simulink model "momentumBasedFlight"  (R2023b)
settings: Solver=VariableStepAuto  StartTime=0.0  StopTime=Config.simulationTime  RelTol=1e-3
InitFcn:
  | cd(fileparts(which(bdroot)));
  | initMomentumBasedFlight;
StopFcn:
  | cd(fileparts(which(bdroot)));
  | stopMomentumBasedFlight;
undefined symbols (not defined in the file or in its folder): aero_config, biasVectorConstraint_feet, Config, confVisualizer, ConstraintMatrix_feet, DiscIntNeverNeededParam, frameNames, Frames, jets_config, robot_config
libraries: WBToolboxLibrary x82, momentum_flight_control_v1 x1, deeplib x1, mwbs_robotDynamicsWithContacts_lib x1
(part 3 of 3)

== system momentumBasedFlight/iRonCub/Forward Dynamics/jetsDyn/Simulink Function2 ==
  simFunc_getWorldTransformJet3Frame : TriggerPort  TriggerType=function-call  IsSimulinkFunction=on  FunctionName=simFunc_getWorldTransformJet3Frame  FunctionVisibility=scoped  VariantControl=(inherit)
  ForwardKinematics : WBToolboxLibrary/Model/Kinematics/ForwardKinematics  frameName=Frames.JET3_FRAME
      settings: SourceProductName=WholeBodyToolbox
  basePose : ArgIn  DisableCoverage=on  PortDimensions=[4,4]  ArgumentName=basePose
  jointPosition : ArgIn  Port=2  PortDimensions=[robot_config.N_DOF,1]  ArgumentName=jointPosition
  w_H_jet3Frame : ArgOut  DisableCoverage=on  PortDimensions=[4,4]  ArgumentName=w_H_jet3Frame
  wires:
  ForwardKinematics/1 -> w_H_jet3Frame/1
  jointPosition/1 -> ForwardKinematics/2
  basePose/1 -> ForwardKinematics/1

== system momentumBasedFlight/iRonCub/Forward Dynamics/jetsDyn/Simulink Function3 ==
  simFunc_getWorldTransformJet4Frame : TriggerPort  TriggerType=function-call  IsSimulinkFunction=on  FunctionName=simFunc_getWorldTransformJet4Frame  FunctionVisibility=scoped  VariantControl=(inherit)
  ForwardKinematics : WBToolboxLibrary/Model/Kinematics/ForwardKinematics  frameName=Frames.JET4_FRAME
      settings: SourceProductName=WholeBodyToolbox
  basePose : ArgIn  DisableCoverage=on  PortDimensions=[4,4]  ArgumentName=basePose
  jointPosition : ArgIn  Port=2  PortDimensions=[robot_config.N_DOF,1]  ArgumentName=jointPosition
  w_H_jet4Frame : ArgOut  DisableCoverage=on  PortDimensions=[4,4]  ArgumentName=w_H_jet4Frame
  wires:
  basePose/1 -> ForwardKinematics/1
  jointPosition/1 -> ForwardKinematics/2
  ForwardKinematics/1 -> w_H_jet4Frame/1

== system momentumBasedFlight/iRonCub/Forward Dynamics/jetsDyn/Simulink Function4 ==
  simFunc_getFrameFreeFloatingJacobianJet2Frame : TriggerPort  TriggerType=function-call  IsSimulinkFunction=on  FunctionName=simFunc_getFrameFreeFloatingJacobianJet2Frame  FunctionVisibility=scoped  VariantControl=(inherit)
  Jacobian Left Foot : WBToolboxLibrary/Model/Jacobians/Jacobian  frameName=Frames.JET2_FRAME
      settings: SourceProductName=WholeBodyToolbox
  basePose : ArgIn  DisableCoverage=on  PortDimensions=[4,4]  ArgumentName=basePose
  jointPosition : ArgIn  Port=2  PortDimensions=[robot_config.N_DOF,1]  ArgumentName=jointPosition
  jacobian : ArgOut  DisableCoverage=on  PortDimensions=[6,6+robot_config.N_DOF]  ArgumentName=jacobian
  wires:
  Jacobian Left Foot/1 -> jacobian/1
  jointPosition/1 -> Jacobian Left Foot/2
  basePose/1 -> Jacobian Left Foot/1

== system momentumBasedFlight/iRonCub/Forward Dynamics/jetsDyn/Simulink Function5 ==
  simFunc_getFrameFreeFloatingJacobianJet3Frame : TriggerPort  TriggerType=function-call  IsSimulinkFunction=on  FunctionName=simFunc_getFrameFreeFloatingJacobianJet3Frame  FunctionVisibility=scoped  VariantControl=(inherit)
  Jacobian Left Foot : WBToolboxLibrary/Model/Jacobians/Jacobian  frameName=Frames.JET3_FRAME
      settings: SourceProductName=WholeBodyToolbox
  basePose : ArgIn  DisableCoverage=on  PortDimensions=[4,4]  ArgumentName=basePose
  jointPosition : ArgIn  Port=2  PortDimensions=[robot_config.N_DOF,1]  ArgumentName=jointPosition
  jacobian : ArgOut  DisableCoverage=on  PortDimensions=[6,6+robot_config.N_DOF]  ArgumentName=jacobian
  wires:
  Jacobian Left Foot/1 -> jacobian/1
  jointPosition/1 -> Jacobian Left Foot/2
  basePose/1 -> Jacobian Left Foot/1

== system momentumBasedFlight/iRonCub/Forward Dynamics/jetsDyn/Simulink Function6 ==
  simFunc_getFrameFreeFloatingJacobianJet4Frame : TriggerPort  TriggerType=function-call  IsSimulinkFunction=on  FunctionName=simFunc_getFrameFreeFloatingJacobianJet4Frame  FunctionVisibility=scoped  VariantControl=(inherit)
  Jacobian Left Foot : WBToolboxLibrary/Model/Jacobians/Jacobian  frameName=Frames.JET4_FRAME
      settings: SourceProductName=WholeBodyToolbox
  basePose : ArgIn  DisableCoverage=on  PortDimensions=[4,4]  ArgumentName=basePose
  jointPosition : ArgIn  Port=2  PortDimensions=[robot_config.N_DOF,1]  ArgumentName=jointPosition
  jacobian : ArgOut  DisableCoverage=on  PortDimensions=[6,6+robot_config.N_DOF]  ArgumentName=jacobian
  wires:
  Jacobian Left Foot/1 -> jacobian/1
  jointPosition/1 -> Jacobian Left Foot/2
  basePose/1 -> Jacobian Left Foot/1

== system momentumBasedFlight/iRonCub/Forward Dynamics/jetsDyn/Simulink Function7 ==
  simFunc_getWorldTransformJet1Frame : TriggerPort  TriggerType=function-call  IsSimulinkFunction=on  FunctionName=simFunc_getWorldTransformJet1Frame  FunctionVisibility=scoped  VariantControl=(inherit)
  ForwardKinematics : WBToolboxLibrary/Model/Kinematics/ForwardKinematics  frameName=Frames.JET1_FRAME
      settings: SourceProductName=WholeBodyToolbox
  basePose : ArgIn  DisableCoverage=on  PortDimensions=[4,4]  ArgumentName=basePose
  jointPosition : ArgIn  Port=2  PortDimensions=[robot_config.N_DOF,1]  ArgumentName=jointPosition
  w_H_jet1Frame : ArgOut  DisableCoverage=on  PortDimensions=[4,4]  ArgumentName=w_H_jet1Frame
  wires:
  basePose/1 -> ForwardKinematics/1
  jointPosition/1 -> ForwardKinematics/2
  ForwardKinematics/1 -> w_H_jet1Frame/1

== system momentumBasedFlight/FLIGHT CONTROLLER (CORE) V3.0/Flight Controller RAL-HUMANOIDS V3.0/Joint Torque Control for Flying/QP torqueControl/QP torqueControl - balancing ==
  H : Inport
  g : Inport  Port=2
  ub : Inport  Port=3
  lb : Inport  Port=4
  AEq : Inport  Port=5
  lbEq : Inport  Port=6
  ubEq : Inport  Port=7
  Enable : EnablePort
  Combine Bounds and Inequalities : MATLAB Function  TreatAsAtomicUnit=on
  MatchSignalSizes : WBToolboxLibrary/Utilities/MatchSignalSizes
      settings: SourceProductName=WholeBodyToolbox
  QP balancing-torqueControl : WBToolboxLibrary/Utilities/QP  lbA=on  ubA=on  lb=off  ub=off  computeObjVal=off  stopIfFails=off
      settings: SourceProductName=WholeBodyToolbox
  QPStatus_balancing : Outport  VectorParamsAs1DForOutWhenUnconnected=off
  QPOutput_balancing : Outport  Port=2  VectorParamsAs1DForOutWhenUnconnected=off
  wires:
  Combine Bounds and Inequalities/3(ubEq_combined) -> QP balancing-torqueControl/5
  Combine Bounds and Inequalities/2(lbEq_combined) -> QP balancing-torqueControl/4
  Combine Bounds and Inequalities/1(AEq_combined) -> QP balancing-torqueControl/3
  ub/1 -> Combine Bounds and Inequalities/5(ub)
  lb/1 -> Combine Bounds and Inequalities/4(lb)
  ubEq/1 -> Combine Bounds and Inequalities/3(ubEq)
  lbEq/1 -> Combine Bounds and Inequalities/2(lbEq)
  AEq/1 -> Combine Bounds and Inequalities/1(AEq)
  g/1 -> QP balancing-torqueControl/2, MatchSignalSizes/1
  H/1 -> QP balancing-torqueControl/1
  QP balancing-torqueControl/1 -> MatchSignalSizes/2
  MatchSignalSizes/1 -> QPOutput_balancing/1
  QP balancing-torqueControl/2 -> QPStatus_balancing/1

== system momentumBasedFlight/FLIGHT CONTROLLER (CORE) V3.0/Flight Controller RAL-HUMANOIDS V3.0/Joint Torque Control for Flying/QP torqueControl/QP torqueControl - flight ==
  H : Inport
  g : Inport  Port=2
  ub : Inport  Port=3
  lb : Inport  Port=4
  Enable : EnablePort
  Constant : Constant  Value=eye(Config.N_DOF)
  MatchSignalSizes : WBToolboxLibrary/Utilities/MatchSignalSizes
      settings: SourceProductName=WholeBodyToolbox
  QP flight-torqueControl : WBToolboxLibrary/Utilities/QP  lbA=on  ubA=on  lb=off  ub=off  computeObjVal=off  stopIfFails=off
      settings: SourceProductName=WholeBodyToolbox
  QPStatus_flight : Outport  VectorParamsAs1DForOutWhenUnconnected=off
  QPOutput_flight : Outport  Port=2  VectorParamsAs1DForOutWhenUnconnected=off
  wires:
  ub/1 -> QP flight-torqueControl/5
  g/1 -> MatchSignalSizes/1, QP flight-torqueControl/2
  H/1 -> QP flight-torqueControl/1
  QP flight-torqueControl/1 -> MatchSignalSizes/2
  MatchSignalSizes/1 -> QPOutput_flight/1
  lb/1 -> QP flight-torqueControl/4
  QP flight-torqueControl/2 -> QPStatus_flight/1
  Constant/1 -> QP flight-torqueControl/3

== system momentumBasedFlight/FLIGHT CONTROLLER (CORE) V3.0/Flight Controller RAL-HUMANOIDS V3.0/Joint Torque Control for Flying/QP torqueControl/Select QP torqueControl Output ==
  QPStatus_balancing : Inport
  QPOutput_balancing : Inport  Port=2
  feetContactIsActive : Inport  Port=3
  QPStatus_flight : Inport  Port=4
  QPOutput_flight : Inport  Port=5
  Demux : Demux  Outputs=[12;Config.N_DOF]
  Switch : Switch  Criteria=u2 > Threshold  SaturateOnIntegerOverflow=off  InputSameDT=off
  Switch1 : Switch  Criteria=u2 > Threshold  SaturateOnIntegerOverflow=off  InputSameDT=off
  contactForces_QP : Terminator
  jointTorques_star : Outport  VectorParamsAs1DForOutWhenUnconnected=off
  exitFlagQP_torqueControl : Outport  Port=2  VectorParamsAs1DForOutWhenUnconnected=off
  wires:
  Demux/2 -> Switch1/1
  Demux/1 -> contactForces_QP/1
  QPOutput_flight/1 -> Switch1/3
  QPOutput_balancing/1 -> Demux/1
  Switch/1 -> exitFlagQP_torqueControl/1
  QPStatus_flight/1 -> Switch/3
  QPStatus_balancing/1 -> Switch/1
  feetContactIsActive/1 -> Switch/2, Switch1/2
  Switch1/1 -> jointTorques_star/1

== system momentumBasedFlight/FLIGHT CONTROLLER (CORE) V3.0/Flight Controller RAL-HUMANOIDS V3.0/Momentum Control for Flying/QP Solver and Integrate Contact Forces Derivative/Integrate the Contact Forces Derivative ==
  contactForcesDot_star : Inport
  contactForces : Inport  Port=2
  feetContactIsActive : Inport  Port=3
  Discrete-Time Integrator1 : DiscreteIntegrator  ExternalReset=either  InitialConditionSource=external  InitialCondition=zeros(6,1)  SampleTime=Config.tStep  ICPrevOutput=DiscIntNeverNeededParam  ICPrevScaledInput=DiscIntNeverNeededParam
  Select Integrator Initial Condition : MATLAB Function  TreatAsAtomicUnit=on
  deadZone : Subsystem
  contactForces_star : Outport  VectorParamsAs1DForOutWhenUnconnected=off
  tag scope: contactForcesDot_star=global
  wires:
  Select Integrator Initial Condition/1(contactForces_0) -> Discrete-Time Integrator1/3
  feetContactIsActive/1 -> Discrete-Time Integrator1/2, Select Integrator Initial Condition/1(feetContactIsActive)
  contactForces/1 -> Select Integrator Initial Condition/2(contactForces)
  deadZone/1(u_cut) -> Discrete-Time Integrator1/1
  contactForcesDot_star/1 -> [contactForcesDot_star], deadZone/1(u)
  Discrete-Time Integrator1/1 -> contactForces_star/1

== system momentumBasedFlight/FLIGHT CONTROLLER (CORE) V3.0/Flight Controller RAL-HUMANOIDS V3.0/Momentum Control for Flying/QP Solver and Integrate Contact Forces Derivative/QP momentumControl ==
  HessianMatrixQP : Inport
  gVectorQP : Inport  Port=2
  lowerBoundQP : Inport  Port=3
  upperBoundQP : Inport  Port=4
  feetContactIsActive : Inport  Port=5
  NOT : Logic  Operator=NOT  IconShape=distinctive  AllPortsSameDT=off  OutDataTypeStr=boolean
  Process QP Inputs Momentum Control : MATLAB Function  TreatAsAtomicUnit=on
  QP momentumControl - balancing : Subsystem  TreatAsAtomicUnit=on
  QP momentumControl - flight : Subsystem  TreatAsAtomicUnit=on
  Select QP momentumControl Output : Subsystem
  jetsIntensitiesDot_star : Outport  VectorParamsAs1DForOutWhenUnconnected=off
  contactForcesDot_star : Outport  Port=2  VectorParamsAs1DForOutWhenUnconnected=off
  jointVel_star : Outport  Port=3  VectorParamsAs1DForOutWhenUnconnected=off
  exitFlagQP_momentumControl : Outport  Port=4  VectorParamsAs1DForOutWhenUnconnected=off
  wires:
  QP momentumControl - flight/2(QPOutput_flight) -> Select QP momentumControl Output/5(QPOutput_flight)
  QP momentumControl - flight/1(QPStatus_flight) -> Select QP momentumControl Output/4(QPStatus_flight)
  QP momentumControl - balancing/2(QPOutput_balancing) -> Select QP momentumControl Output/2(QPOutput_balancing)
  QP momentumControl - balancing/1(QPStatus_balancing) -> Select QP momentumControl Output/1(QPStatus_balancing)
  Select QP momentumControl Output/4(exitFlagQP_momentumControl) -> exitFlagQP_momentumControl/1
  NOT/1 -> QP momentumControl - flight/Enable
  Process QP Inputs Momentum Control/8(lb_flight) -> QP momentumControl - flight/4(lb)
  Process QP Inputs Momentum Control/7(ub_flight) -> QP momentumControl - flight/3(ub)
  Process QP Inputs Momentum Control/4(lb_balancing) -> QP momentumControl - balancing/4(lb)
  Process QP Inputs Momentum Control/3(ub_balancing) -> QP momentumControl - balancing/3(ub)
  Process QP Inputs Momentum Control/6(g_flight) -> QP momentumControl - flight/2(g)
  Process QP Inputs Momentum Control/5(H_flight) -> QP momentumControl - flight/1(H)
  Process QP Inputs Momentum Control/2(g_balancing) -> QP momentumControl - balancing/2(g)
  Process QP Inputs Momentum Control/1(H_balancing) -> QP momentumControl - balancing/1(H)
  Select QP momentumControl Output/2(contactForcesDot_star) -> contactForcesDot_star/1
  Select QP momentumControl Output/3(jointVel_star) -> jointVel_star/1
  Select QP momentumControl Output/1(jetsIntensitiesDot_star) -> jetsIntensitiesDot_star/1
  HessianMatrixQP/1 -> Process QP Inputs Momentum Control/1(HessianMatrixQP)
  upperBoundQP/1 -> Process QP Inputs Momentum Control/4(upperBoundQP)
  feetContactIsActive/1 -> QP momentumControl - balancing/Enable, NOT/1, Select QP momentumControl Output/3(feetContactIsActive)
  lowerBoundQP/1 -> Process QP Inputs Momentum Control/3(lowerBoundQP)
  gVectorQP/1 -> Process QP Inputs Momentum Control/2(gVectorQP)

== system momentumBasedFlight/FLIGHT CONTROLLER (CORE) V3.0/Flight Controller RAL-HUMANOIDS V3.0/Momentum Control for Flying/QP Solver and Integrate Contact Forces Derivative/Integrate the Contact Forces Derivative/deadZone ==
  u : Inport
  Constant : Constant  Value=Config.sat.deadZoneThreshold
  Deadzone Function : MATLAB Function  TreatAsAtomicUnit=on
  u_cut : Outport  VectorParamsAs1DForOutWhenUnconnected=off
  wires:
  Constant/1 -> Deadzone Function/2(thr)
  u/1 -> Deadzone Function/1(u)
  Deadzone Function/1(y) -> u_cut/1

== system momentumBasedFlight/FLIGHT CONTROLLER (CORE) V3.0/Flight Controller RAL-HUMANOIDS V3.0/Momentum Control for Flying/QP Solver and Integrate Contact Forces Derivative/QP momentumControl/QP momentumControl - balancing ==
  H : Inport
  g : Inport  Port=2
  ub : Inport  Port=3
  lb : Inport  Port=4
  Enable : EnablePort
  Constant : Constant  Value=eye(Config.N_DOF + 12 + 4)
  MatchSignalSizes : WBToolboxLibrary/Utilities/MatchSignalSizes
      settings: SourceProductName=WholeBodyToolbox
  QP : WBToolboxLibrary/Utilities/QP  lbA=on  ubA=on  lb=off  ub=off  computeObjVal=off  stopIfFails=off
      settings: SourceProductName=WholeBodyToolbox
  QPStatus_balancing : Outport  VectorParamsAs1DForOutWhenUnconnected=off
  QPOutput_balancing : Outport  Port=2  VectorParamsAs1DForOutWhenUnconnected=off
  wires:
  ub/1 -> QP/5
  QP/1 -> MatchSignalSizes/2
  MatchSignalSizes/1 -> QPOutput_balancing/1
  QP/2 -> QPStatus_balancing/1
  H/1 -> QP/1
  g/1 -> MatchSignalSizes/1, QP/2
  lb/1 -> QP/4
  Constant/1 -> QP/3

== system momentumBasedFlight/FLIGHT CONTROLLER (CORE) V3.0/Flight Controller RAL-HUMANOIDS V3.0/Momentum Control for Flying/QP Solver and Integrate Contact Forces Derivative/QP momentumControl/QP momentumControl - flight ==
  H : Inport
  g : Inport  Port=2
  ub : Inport  Port=3
  lb : Inport  Port=4
  Enable : EnablePort
  Constant : Constant  Value=eye(Config.N_DOF + 4)
  MatchSignalSizes : WBToolboxLibrary/Utilities/MatchSignalSizes
      settings: SourceProductName=WholeBodyToolbox
  QP flight-momentumControl : WBToolboxLibrary/Utilities/QP  lbA=on  ubA=on  lb=off  ub=off  computeObjVal=off  stopIfFails=off
      settings: SourceProductName=WholeBodyToolbox
  QPStatus_flight : Outport  VectorParamsAs1DForOutWhenUnconnected=off
  QPOutput_flight : Outport  Port=2  VectorParamsAs1DForOutWhenUnconnected=off
  wires:
  ub/1 -> QP flight-momentumControl/5
  g/1 -> MatchSignalSizes/1, QP flight-momentumControl/2
  H/1 -> QP flight-momentumControl/1
  QP flight-momentumControl/1 -> MatchSignalSizes/2
  MatchSignalSizes/1 -> QPOutput_flight/1
  lb/1 -> QP flight-momentumControl/4
  QP flight-momentumControl/2 -> QPStatus_flight/1
  Constant/1 -> QP flight-momentumControl/3

== system momentumBasedFlight/FLIGHT CONTROLLER (CORE) V3.0/Flight Controller RAL-HUMANOIDS V3.0/Momentum Control for Flying/QP Solver and Integrate Contact Forces Derivative/QP momentumControl/Select QP momentumControl Output ==
  QPStatus_balancing : Inport
  QPOutput_balancing : Inport  Port=2
  feetContactIsActive : Inport  Port=3
  QPStatus_flight : Inport  Port=4
  QPOutput_flight : Inport  Port=5
  Constant : Constant  Value=zeros(12,1)
  Demux : Demux  Outputs=[4;12;Config.N_DOF]
  Demux1 : Demux  Outputs=[4;Config.N_DOF]
  Switch{,1..3} (4 alike) : Switch  Criteria=u2 > Threshold  SaturateOnIntegerOverflow=off  InputSameDT=off
  jetsIntensitiesDot_star : Outport  VectorParamsAs1DForOutWhenUnconnected=off
  contactForcesDot_star : Outport  Port=2  VectorParamsAs1DForOutWhenUnconnected=off
  jointVel_star : Outport  Port=3  VectorParamsAs1DForOutWhenUnconnected=off
  exitFlagQP_momentumControl : Outport  Port=4  VectorParamsAs1DForOutWhenUnconnected=off
  wires:
  Demux1/2 -> Switch3/3
  Demux/3 -> Switch3/1
  Constant/1 -> Switch2/3
  Demux/2 -> Switch2/1
  Demux1/1 -> Switch1/3
  Demux/1 -> Switch1/1
  QPOutput_flight/1 -> Demux1/1
  QPOutput_balancing/1 -> Demux/1
  Switch/1 -> exitFlagQP_momentumControl/1
  QPStatus_flight/1 -> Switch/3
  QPStatus_balancing/1 -> Switch/1
  feetContactIsActive/1 -> Switch/2, Switch1/2, Switch2/2, Switch3/2
  Switch3/1 -> jointVel_star/1
  Switch1/1 -> jetsIntensitiesDot_star/1
  Switch2/1 -> contactForcesDot_star/1

== matlab function momentumBasedFlight/FLIGHT CONTROLLER (CORE) V3.0/Jets Control/Feedback linearization/MATLAB Function ==
  data: jets input; jets_dot input; jets_dot_des input; throttle output size=[4,1]; Config parameter; error output; integral_err input
function [throttle, error]  = fl_jet_control(jets, jets_dot, jets_dot_des, Config, integral_err)

[throttle, error]  = fl_jet_control(jets, jets_dot, jets_dot_des, Config, integral_err);
end

== matlab function momentumBasedFlight/FLIGHT CONTROLLER (CORE) V3.0/Flight Controller RAL-HUMANOIDS V3.0/Joint Torque Control for Flying/QP torqueControl/Process QP Inputs Torque Control ==
  data: HessianMatrixQP input; H_balancing output; gVectorQP input; InequalityConstrMatrix input; biasVectorInequalityConstr input; g_balancing output; ub_balancing output; lb_balancing output; Aeq_balancing output; lbEq_balancing output; ubEq_balancing output; H_flight output; g_flight output; ub_flight output; lb_flight output; jointTorquesSaturation input; Config parameter
function [H_balancing,g_balancing,ub_balancing,lb_balancing,Aeq_balancing,lbEq_balancing,ubEq_balancing, ...
          H_flight,g_flight,ub_flight,lb_flight] = processQPinputTorqueControlFCN ...
                                                       (HessianMatrixQP,gVectorQP,InequalityConstrMatrix, ...
                                                        biasVectorInequalityConstr,jointTorquesSaturation,Config)   
   
[H_balancing,g_balancing,ub_balancing,lb_balancing,Aeq_balancing,lbEq_balancing,ubEq_balancing, ...
          H_flight,g_flight,ub_flight,lb_flight] = iRonCubLib_v1.processQPinputTorqueControl ...
                                                       (HessianMatrixQP,gVectorQP,InequalityConstrMatrix, ...
                                                        biasVectorInequalityConstr,jointTorquesSaturation,Config);     
end

== matlab function momentumBasedFlight/FLIGHT CONTROLLER (CORE) V3.0/Flight Controller RAL-HUMANOIDS V3.0/Joint Torque Control for Flying/QP torqueControl/QP torqueControl - balancing/Combine Bounds and Inequalities ==
  data: AEq input; AEq_combined output; lbEq input; ubEq input; lb input; ub input; lbEq_combined output; ubEq_combined output
function [AEq_combined,lbEq_combined,ubEq_combined] = combineInputBoundsAndInequalitiesQPFCN(AEq,lbEq,ubEq,lb,ub)

   [AEq_combined,lbEq_combined,ubEq_combined] = iRonCubLib_v1.combineInputBoundsAndInequalitiesQP(AEq,lbEq,ubEq,lb,ub);
end

== matlab function momentumBasedFlight/FLIGHT CONTROLLER (CORE) V3.0/Jets Control/extendedKalmanFilter4jets/EKF_jet1/EKF  ==
  data: x input; input input; measurement input; xDot output; P input; Config parameter; Pdot output
function [xDot, Pdot] = extendedKalmanFilterFNC(x, input, measurement, P, Config)

[xDot, Pdot] = extKalmanFilter(x, input, Config.jetC_P100, P, measurement, Config);

== matlab function momentumBasedFlight/FLIGHT CONTROLLER (CORE) V3.0/Flight Controller RAL-HUMANOIDS V3.0/Joint Torque Control for Flying/torqueControlFCN ==
  data: M input; h input; J_jets input; J_LFoot input; J_RFoot input; JDot_LFoot_nu input; JDot_RFoot_nu input; J_aeroForces input; w_H_LFoot input; w_H_RFoot input; matrixOfJetsAxes input; ConstraintsMatrix_feet input; biasVectorConstraint_feet input; jetsIntensities input; stateVel input; jointVel_star input; contactForces_star input; KI_torqueControl input; KP_torqueControl input; feetContactIsActive input; activateEqConstrTorqueControl input; robotIsLanded input; aerodynamic_forces input; jointPos_err input; Hessian output; Config parameter; gradient output; ConstraintMatrix_inequality output; biasVectorConstraint_inequality output; jointVel_err output; aero_config parameter
function [Hessian, gradient, ConstraintMatrix_inequality, biasVectorConstraint_inequality, jointVel_err] =  ... 
             aeroFlyingTorqueControlFCN(M, h, J_jets, J_LFoot, J_RFoot, JDot_LFoot_nu, JDot_RFoot_nu, J_aeroForces, w_H_LFoot, w_H_RFoot, matrixOfJetsAxes, ...
                                        ConstraintsMatrix_feet, biasVectorConstraint_feet, jetsIntensities, stateVel, jointVel_star, contactForces_star, ...
                                        KI_torqueControl, KP_torqueControl, feetContactIsActive, activateEqConstrTorqueControl, robotIsLanded, aerodynamic_forces, jointPos_err, Config, aero_config)
                                      
    [Hessian, gradient, ConstraintMatrix_inequality, biasVectorConstraint_inequality, jointVel_err] =  ... 
        aeroFlyingTorqueControl(M, h, J_jets, J_LFoot, J_RFoot, JDot_LFoot_nu, JDot_RFoot_nu, J_aeroForces, w_H_LFoot, w_H_RFoot, matrixOfJetsAxes, ...
                                ConstraintsMatrix_feet, biasVectorConstraint_feet, jetsIntensities, stateVel, jointVel_star, contactForces_star, ...
                                KI_torqueControl, KP_torqueControl, feetContactIsActive, activateEqConstrTorqueControl, robotIsLanded, aerodynamic_forces, jointPos_err, aero_config, Config);           
end

== matlab function momentumBasedFlight/FLIGHT CONTROLLER (CORE) V3.0/Flight Controller RAL-HUMANOIDS V3.0/Momentum Control for Flying/Momentum Control/Aerodynamic Flying Controller Momentum FCN  ==
  data: jointPos input; w_baseTwist input; jetsIntensities input; J_jets input; J_CoM input; J_LFoot input; J_RFoot input; posCoM input; w_R_b input; w_H_LFoot input; w_H_RFoot input; matrixOfJetsAxes input; matrixOfJetsArms input; matrixOfAeroArms input; J_aeroForces input; w_I_c input; L input; M input; CMM input; pos_vel_acc_jerk_CoM_des input; rot_vel_acc_jerk_base_des input size=[3,6]; jointPos_des input; KP_momentum input; KD_momentum input; KP_postural input; feetContactIsActive input; decreaseMaxFootVerticalForce input; increaseMinFootVerticalForce input; robotIsLanded input; HessianMatrixQP output; gVectorQP output; lowerBoundQP output; upperBoundQP output; L_des output; LDot_estimated output; verifyAngMomAndInertia output; contactForces_hat input; aerodynamic_forces input; Config parameter; velCoM output; aero_config parameter
function [HessianMatrixQP, gVectorQP, lowerBoundQP, upperBoundQP, L_des, LDot_estimated, verifyAngMomAndInertia, velCoM] = ...
             aeroFlyingMomentumControlFCN(jointPos, w_baseTwist, jetsIntensities, J_jets, J_CoM, J_LFoot, J_RFoot, posCoM, w_R_b, w_H_LFoot, w_H_RFoot, ...
                                          matrixOfJetsAxes, matrixOfJetsArms, matrixOfAeroArms, J_aeroForces, w_I_c, L, M, CMM, pos_vel_acc_jerk_CoM_des, ....
                                          rot_vel_acc_jerk_base_des, jointPos_des, KP_momentum, KD_momentum, KP_postural, feetContactIsActive, ...
                                          decreaseMaxFootVerticalForce, increaseMinFootVerticalForce, robotIsLanded, contactForces_hat, aerodynamic_forces, Config, aero_config)
                               
    [HessianMatrixQP, gVectorQP, lowerBoundQP, upperBoundQP, L_des, LDot_estimated, verifyAngMomAndInertia, velCoM] = ...
        aeroFlyingMomentumControl(jointPos, w_baseTwist, jetsIntensities, J_jets, J_CoM, J_LFoot, J_RFoot, posCoM, w_R_b, w_H_LFoot, w_H_RFoot, ...
                                  matrixOfJetsAxes, matrixOfJetsArms, matrixOfAeroArms, J_aeroForces, w_I_c, L, M, CMM, pos_vel_acc_jerk_CoM_des, ....
                                  rot_vel_acc_jerk_base_des, jointPos_des, KP_momentum, KD_momentum, KP_postural, feetContactIsActive, ...
                                  decreaseMaxFootVerticalForce, increaseMinFootVerticalForce, robotIsLanded, contactForces_hat, aerodynamic_forces, aero_config, Config);
end

== matlab function momentumBasedFlight/FLIGHT CONTROLLER (CORE) V3.0/Jets Control/extendedKalmanFilter4jets/EKF_jet1/splitVector ==
  data: x input; x1 output; x2 output
function [x1, x2] = fcn(x)
x1 = x(1);
x2 = x(2);

== matlab function momentumBasedFlight/Visualizer/Task and Base Frame Kinematics/Get RPY error norm ==
  data: rot_err input; rotErr_norm output
function rotErr_norm = normFCN(rot_err)

rotErr_norm = norm(rot_err);

end

== matlab function momentumBasedFlight/FLIGHT CONTROLLER (CORE) V3.0/Flight Controller RAL-HUMANOIDS V3.0/Momentum Control for Flying/QP Solver and Integrate Contact Forces Derivative/Integrate the Contact Forces Derivative/Select Integrator Initial Condition ==
  data: feetContactIsActive input; contactForces input; contactForces_0 output
function contactForces_0 = selectInitContactForcesFCN(feetContactIsActive, contactForces)

    contactForces_0 = iRonCubLib_v1.selectInitContactForces(feetContactIsActive, contactForces);
end

== matlab function momentumBasedFlight/FLIGHT CONTROLLER (CORE) V3.0/Jets Control/extendedKalmanFilter4jets/EKF_jet2/EKF  ==
  data: x input; input input; measurement input; xDot output; P input; Config parameter; Pdot output
function [xDot, Pdot] = extendedKalmanFilterFNC(x, input, measurement, P, Config)

[xDot, Pdot] = extKalmanFilter(x, input, Config.jetC_P100, P, measurement, Config);

== matlab function momentumBasedFlight/FLIGHT CONTROLLER (CORE) V3.0/Dynamics and Kinematics/Kinematic Quantities/Compute Aerodynamic Forces Homogeneous Transform/Aero Transforms ==
  data: w_H_LinkFrames input; posCoM input; matrixOfLinkCoMTransform output; Config parameter; aero_config parameter
function matrixOfLinkCoMTransform = computeMatrixOfLinkCoMTransformFCN(w_H_LinkFrames, posCoM, Config, aero_config)

    matrixOfLinkCoMTransform = computeMatrixOfLinkCoMTransform(w_H_LinkFrames, posCoM, aero_config, Config);
end

== matlab function momentumBasedFlight/FLIGHT CONTROLLER (CORE) V3.0/Get System State/Change Contact Forces Representation/Change Contact Forces Representation ==
  data: contactForces_WBD input; mixed_f_l_sole output; w_R_l_sole input; w_R_r_sole input; mixed_f_r_sole output
function [mixed_f_l_sole, mixed_f_r_sole] = fromBodyFrameToMixed_contactForcesFCN(contactForces_WBD, w_R_l_sole, w_R_r_sole)

    [mixed_f_l_sole, mixed_f_r_sole] = iRonCubLib_v1.fromBodyFrameToMixed_contactForces(contactForces_WBD, w_R_l_sole, w_R_r_sole);
end

== matlab function momentumBasedFlight/Visualizer/Task and Base Frame Kinematics/Get RPY from rotation matrix ==
  data: w_R_b input; rollPitchYaw output
function rollPitchYaw = rollPitchYawFromRotationFCN(w_R_b)

rollPitchYaw = wbc.rollPitchYawFromRotation(w_R_b);

end

== matlab function momentumBasedFlight/Visualizer/Task and Base Frame Kinematics/Get RPY from rotation matrix  ==
  data: w_R_b input; rollPitchYaw output
function rollPitchYaw = rollPitchYawFromRotationFCN(w_R_b)

rollPitchYaw = wbc.rollPitchYawFromRotation(w_R_b);

end

== matlab function momentumBasedFlight/Visualizer/Task and Base Frame Kinematics/MATLAB Function1 ==
  data: RPY_Corr output; rollPitchYaw input
function RPY_Corr = correctYawAngleFCN(rollPitchYaw)

    RPY_Corr = correctYawAngle(rollPitchYaw);

end

== matlab function momentumBasedFlight/FLIGHT CONTROLLER (CORE) V3.0/Jets Control/extendedKalmanFilter4jets/EKF_jet2/splitVector ==
  data: x input; x1 output; x2 output
function [x1, x2] = fcn(x)
x1 = x(1);
x2 = x(2);

== matlab function momentumBasedFlight/FLIGHT CONTROLLER (CORE) V3.0/Jets Control/extendedKalmanFilter4jets/EKF_jet3/EKF  ==
  data: x input; input input; measurement input; xDot output; P input; Config parameter; Pdot output
function [xDot, Pdot] = extendedKalmanFilterFNC(x, input, measurement, P, Config)

[xDot, Pdot] = extKalmanFilter(x, input, Config.jetC_P220, P, measurement, Config);

== matlab function momentumBasedFlight/Visualizer/Task and Base Frame Kinematics/MATLAB Function2 ==
  data: RPY_Corr output; rollPitchYaw input
function RPY_Corr = correctYawAngleFCN(rollPitchYaw)

    RPY_Corr = correctYawAngle(rollPitchYaw);

end

== matlab function momentumBasedFlight/FLIGHT CONTROLLER (CORE) V3.0/Jets Control/extendedKalmanFilter4jets/EKF_jet3/splitVector ==
  data: x input; x1 output; x2 output
function [x1, x2] = fcn(x)
x1 = x(1);
x2 = x(2);

== matlab function momentumBasedFlight/Visualizer/Task and Base Frame Kinematics/MATLAB Function3 ==
  data: RPY_Corr output; rollPitchYaw input
function RPY_Corr = correctYawAngleFCN(rollPitchYaw)

    RPY_Corr = correctYawAngle(rollPitchYaw);

end

== matlab function momentumBasedFlight/iRonCub/Forward Dynamics/jetsDyn/MATLAB Function ==
  data: u input; u1 output; u2 output; u3 output; u4 output
function [u1, u2, u3, u4] = splitVec(u)
u1 = u(1);
u2 = u(2);
u3 = u(3);
u4 = u(4);

== matlab function momentumBasedFlight/FLIGHT CONTROLLER (CORE) V3.0/Jets Control/extendedKalmanFilter4jets/EKF_jet4/EKF  ==
  data: x input; input input; measurement input; xDot output; P input; Config parameter; Pdot output
function [xDot, Pdot] = extendedKalmanFilterFNC(x, input, measurement, P, Config)

[xDot, Pdot] = extKalmanFilter(x, input, Config.jetC_P220, P, measurement, Config);

== matlab function momentumBasedFlight/FLIGHT CONTROLLER (CORE) V3.0/Jets Control/extendedKalmanFilter4jets/EKF_jet4/splitVector ==
  data: x input; x1 output; x2 output
function [x1, x2] = fcn(x)
x1 = x(1);
x2 = x(2);

== matlab function momentumBasedFlight/FLIGHT CONTROLLER (CORE) V3.0/Dynamics and Kinematics/Dynamic Quantities/Compute Centroidal Inertia/Compute Centroidal Inertia ==
  data: M input; w_I_c output; posCoM input; posBase input
function w_I_c = getCentrInertiaFCN(M, posCoM, posBase)

    w_I_c = iRonCubLib_v1.getCentrInertia(M, posCoM, posBase);
end

== matlab function momentumBasedFlight/FLIGHT CONTROLLER (CORE) V3.0/Dynamics and Kinematics/Kinematic Quantities/Compute Thrusts Axes and Arms/Thrust Axes and Arms ==
  data: w_H_J1 input; matrixOfJetsAxes output; w_H_J2 input; w_H_J3 input; w_H_J4 input; posCoM input; matrixOfJetsArms output; Config parameter
function [matrixOfJetsAxes, matrixOfJetsArms] = computeJetsAxesAndArmsFCN(w_H_J1, w_H_J2, w_H_J3, w_H_J4, posCoM, Config)

    [matrixOfJetsAxes, matrixOfJetsArms] = iRonCubLib_v1.computeJetsAxesAndArms(w_H_J1, w_H_J2, w_H_J3, w_H_J4, posCoM, Config);
end

== matlab function momentumBasedFlight/FLIGHT CONTROLLER (CORE) V3.0/Dynamics and Kinematics/Kinematic Quantities/Compute Aerodynamic Forces Arms/Thrust Axes and Arms ==
  data: w_H_LinkFrames input; posCoM input; matrixOfAeroArms output; Config parameter; aero_config parameter
function matrixOfAeroArms = computeAeroArmsFCN(w_H_LinkFrames, posCoM, Config, aero_config)

    matrixOfAeroArms = computeAeroArms(w_H_LinkFrames, posCoM, aero_config, Config);
end

== matlab function momentumBasedFlight/FLIGHT CONTROLLER (CORE) V3.0/Dynamics and Kinematics/Kinematic Quantities/Compute Aerodynamic Forces Jacobians/compute matrix of link CoM Jacobians ==
  data: w_H_b input; linkFrameJacobians input; J_aeroForces output; aero_config parameter
function J_aeroForces = computeMatrixOfLinkCoMJacobians(w_H_b, linkFrameJacobians, aero_config)

    J_aeroForces = computeMatrixOfLinkCoMJacobians(w_H_b, linkFrameJacobians, aero_config);

end

== matlab function momentumBasedFlight/Visualizer/Aerodynamics/Vectors norm ==
  data: aeroForces input; aeroForcesNorms output
function aeroForcesNorms = computeAeroForcesNorms(aeroForces)

    aeroForcesNorms = zeros(size(aeroForces,2),1);
    
    for i = 1 : length(aeroForcesNorms)
        aeroForcesNorms(i) = norm(aeroForces(:,i));
    end

end

== matlab function momentumBasedFlight/Wind Profile Generator/Wind Velocity Profile Generator ==
  data: maxWindVelocity input; windVelocity output; time input; Config parameter
function windVelocity = generateWindVelocityFCN(maxWindVelocity, time, Config)
    
    windVelocity = generateWindVelocity(maxWindVelocity, time, Config);

end

== matlab function momentumBasedFlight/iRonCub/Forward Dynamics/AerodyNNamics/Compute AerodyNNamics Inputs ==
  data: w_H_b input; base_velocity input; joints_position input; windSpeed input; b_relWindDir output; jointPosDeg output
function [b_relWindDir, jointPosDeg] = computeAeroNetInputsFcn(w_H_b, base_velocity, joints_position, windSpeed)
    
    [b_relWindDir, jointPosDeg] = computeAeroNetInputs(w_H_b, base_velocity, joints_position, windSpeed);

end

== matlab function momentumBasedFlight/iRonCub/Forward Dynamics/AerodyNNamics/Rotate Output from aerodynamic to world frame ==
  data: w_H_b input; aerodynamicForceAreas input; w_aerodynamicForceAreas output
function w_aerodynamicForceAreas = transformAeroNetOutputFcn(w_H_b, aerodynamicForceAreas)
    
    w_aerodynamicForceAreas = transformAeroNetOutput(w_H_b, aerodynamicForceAreas);

end

== matlab function momentumBasedFlight/FLIGHT CONTROLLER (CORE) V3.0/JoyStick-flightGUI Commands1/Autopilot ==
  data: time input; joyButtons output; joyAxes output; Config parameter
function [joyButtons,joyAxes] = autopilotFCN(time, Config)

    [joyButtons,joyAxes] = autopilot(time, Config);
end

== matlab function momentumBasedFlight/FLIGHT CONTROLLER (CORE) V3.0/JoyStick-flightGUI Commands1/Replace Joystick with Native GUI ==
  data: gui_input input; joyButtons output; joyAxes output
function [joyButtons,joyAxes] = fromGuiToJoystickFCN(gui_input)

    [joyButtons,joyAxes] = iRonCubLib_v1.fromGuiToJoystick(gui_input);
end

== matlab function momentumBasedFlight/Visualizer/Aerodynamics/Vectors norm1 ==
  data: aeroForces input; aeroForcesNorms output
function aeroForcesNorms = computeAeroForcesNorms(aeroForces)

    aeroForcesNorms = zeros(size(aeroForces,2),1);
    
    for i = 1 : length(aeroForcesNorms)
        aeroForcesNorms(i) = norm(aeroForces(:,i));
    end

end

== matlab function momentumBasedFlight/FLIGHT CONTROLLER (CORE) V3.0/Flight Controller RAL-HUMANOIDS V3.0/Momentum Control for Flying/QP Solver and Integrate Contact Forces Derivative/Integrate the Contact Forces Derivative/deadZone/Deadzone Function ==
  data: u input; y output; thr input
function y = deadZoneFCN(u, thr)

    y = wbc.deadZone(u, thr);
end

== matlab function momentumBasedFlight/FLIGHT CONTROLLER (CORE) V3.0/Flight Controller RAL-HUMANOIDS V3.0/Momentum Control for Flying/QP Solver and Integrate Contact Forces Derivative/QP momentumControl/Process QP Inputs Momentum Control ==
  data: HessianMatrixQP input; H_balancing output; gVectorQP input; lowerBoundQP input; upperBoundQP input; g_balancing output; ub_balancing output; lb_balancing output; H_flight output; g_flight output; ub_flight output; lb_flight output
function [H_balancing,g_balancing,ub_balancing,lb_balancing, ...
          H_flight,g_flight,ub_flight,lb_flight] = processQPinputMomentumControlFCN(HessianMatrixQP,gVectorQP,lowerBoundQP,upperBoundQP) 
      
    [H_balancing,g_balancing,ub_balancing,lb_balancing, ...
        H_flight,g_flight,ub_flight,lb_flight] = iRonCubLib_v1.processQPinputMomentumControl(HessianMatrixQP,gVectorQP,lowerBoundQP,upperBoundQP);
end

== matlab function momentumBasedFlight/FLIGHT CONTROLLER (CORE) V3.0/Flight Controller RAL-HUMANOIDS V3.0/Joint Torque Control for Flying/Torque Derivative Saturation/Saturate Torque Derivative ==
  data: u input; uSat output; u_0 input; tStep input; uDotMax input
function uSat = saturateInputDerivativeFCN(u, u_0, tStep, uDotMax)

    uSat = wbc.saturateInputDerivative(u, u_0, tStep, uDotMax);
end
